simulink model "mtq_allocation_lib"  (R2018b)
settings: Solver=VariableStepAuto  StartTime=0.0  StopTime=10.0  RelTol=1e-3
libraries: control_command_generation_lib x6
settings Model: Creator=Nick's PC  LastModifiedBy=Nick's PC
settings DataIOCC: SaveOutput=off  SaveTime=off

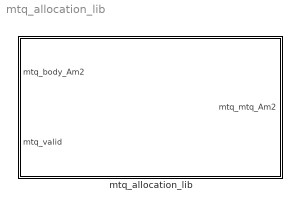
== system mtq_allocation_lib ==
  mtq_allocation_lib : Subsystem

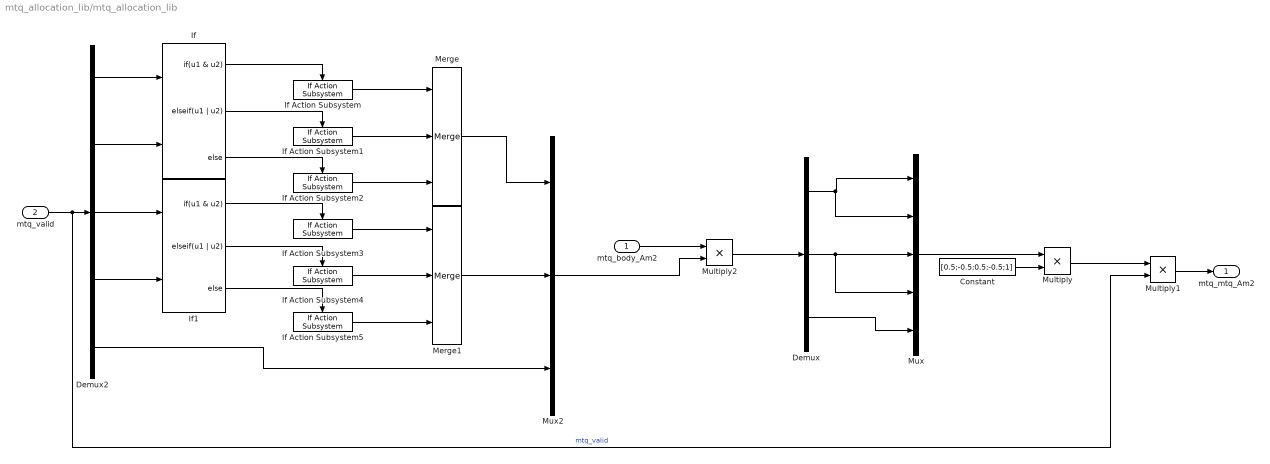
== system mtq_allocation_lib/mtq_allocation_lib ==
  mtq_body_Am2 : Inport
  mtq_valid : Inport  Port=2
  Constant : Constant  Value=[0.5;-0.5;0.5;-0.5;1]
  Demux : Demux  Outputs=3
  Demux2 : Demux  Outputs=5
  If : If  NumInputs=2  IfExpression=u1 & u2  ElseIfExpressions=u1 | u2
  If Action Subsystem : control_command_generation_lib/control_command_generation_lib/mtq_allocation_lib/If Action Subsystem  SystemSampleTime=-1
  If Action Subsystem1 : control_command_generation_lib/control_command_generation_lib/mtq_allocation_lib/If Action Subsystem  SystemSampleTime=-1
      link override Constant: Value=2
  If Action Subsystem2 : control_command_generation_lib/control_command_generation_lib/mtq_allocation_lib/If Action Subsystem  SystemSampleTime=-1
      link override Constant: Value=0
  If Action Subsystem3 : control_command_generation_lib/control_command_generation_lib/mtq_allocation_lib/If Action Subsystem  SystemSampleTime=-1
  If Action Subsystem4 : control_command_generation_lib/control_command_generation_lib/mtq_allocation_lib/If Action Subsystem  SystemSampleTime=-1
      link override Constant: Value=2
  If Action Subsystem5 : control_command_generation_lib/control_command_generation_lib/mtq_allocation_lib/If Action Subsystem  SystemSampleTime=-1
      link override Constant: Value=0
  If1 : If  NumInputs=2  IfExpression=u1 & u2  ElseIfExpressions=u1 | u2
  Merge : Merge  Inputs=3
  Merge1 : Merge  Inputs=3
  Multiply : Product
  Multiply1 : Product
  Multiply2 : Product
  Mux : Mux  Inputs=5
  Mux2 : Mux  Inputs=3
  mtq_mtq_Am2 : Outport
  wires:
  Demux/2 -> Mux/4, Mux/3
  Constant/1 -> Multiply/2
  Demux2/3 -> If1/1
  mtq_valid/1 -> Multiply1/2, Demux2/1  "mtq_valid"
  mtq_body_Am2/1 -> Multiply2/1
  If Action Subsystem4/1 -> Merge1/2
  Multiply2/1 -> Demux/1
  If/1 -> If Action Subsystem/Action
  Mux/1 -> Multiply/1
  Demux/1 -> Mux/2, Mux/1
  Merge1/1 -> Mux2/2
  If1/3 -> If Action Subsystem5/Action
  If1/1 -> If Action Subsystem3/Action
  If Action Subsystem5/1 -> Merge1/3
  Demux/3 -> Mux/5
  Merge/1 -> Mux2/1
  Demux2/4 -> If1/2
  Demux2/5 -> Mux2/3
  If/3 -> If Action Subsystem2/Action
  Multiply/1 -> Multiply1/1
  If Action Subsystem3/1 -> Merge1/1
  Mux2/1 -> Multiply2/2
  If Action Subsystem1/1 -> Merge/2
  If Action Subsystem/1 -> Merge/1
  If/2 -> If Action Subsystem1/Action
  Demux2/2 -> If/2
  If1/2 -> If Action Subsystem4/Action
  If Action Subsystem2/1 -> Merge/3
  Multiply1/1 -> mtq_mtq_Am2/1
  Demux2/1 -> If/1
